simulink model "proj2example"  (R2017a)
settings: Solver=VariableStepAuto  StartTime=0.0  StopTime=inf  RelTol=1e-3
libraries: libraryProject2 x4, realtime_pacer_lib x1
settings Model: Creator=BRAHIMA FANNY  LastModifiedBy=BRAHIMA FANNY

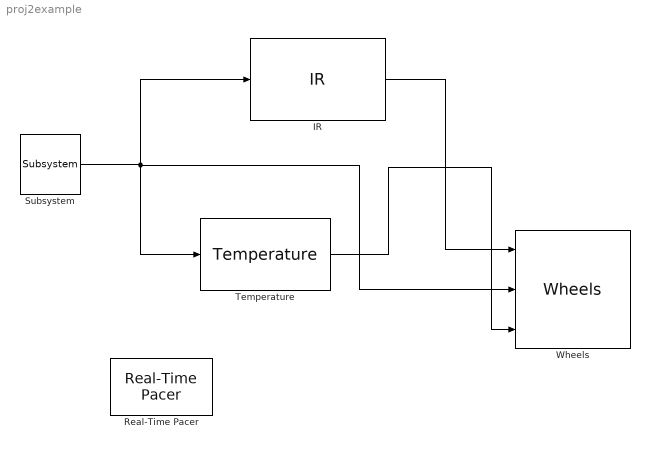
== system proj2example ==
  "IR " : libraryProject2/IR 
  Real-Time Pacer : realtime_pacer_lib/Real-Time Pacer  simTimePerRealTime=.5
  Subsystem : libraryProject2/Subsystem
  Temperature : libraryProject2/Temperature
  Wheels : libraryProject2/Wheels
  wires:
  "IR "/1 -> Wheels/1
  Temperature/1 -> Wheels/3
  Subsystem/1 -> Wheels/2, Temperature/1, "IR "/1
